simulink model "user_test"  (R2020a)
settings: Solver=VariableStepAuto  StartTime=0.0  StopTime=90  RelTol=1e-3
values from neighbouring files (symbols this model uses):
  r = r0    (= 1)    [get_LQR_gain.m]
undefined symbols (not defined in the file or in its folder): DiscIntNeverNeededParam, dt
settings Model: Creator=parke  LastModifiedBy=parke
settings SFSimCC: CustomCodeUndefinedFunction=UseInterfaceOnly

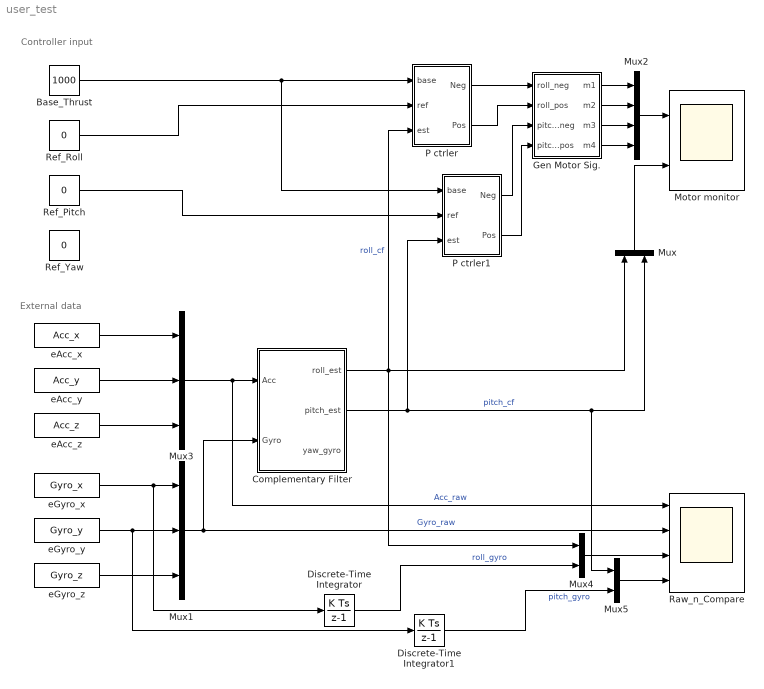
== system user_test ==
  note: External data
  note: Controller input
  Base_Thrust : Constant  Value=1000
  Complementary Filter : Subsystem
  Discrete-Time Integrator : DiscreteIntegrator  gainval=1  SampleTime=dt  ICPrevOutput=DiscIntNeverNeededParam  ICPrevScaledInput=DiscIntNeverNeededParam
  Discrete-Time Integrator1 : DiscreteIntegrator  gainval=1  SampleTime=dt  ICPrevOutput=DiscIntNeverNeededParam  ICPrevScaledInput=DiscIntNeverNeededParam
  Gen Motor Sig. : Subsystem
  Motor monitor : Scope  NumInputPorts=2
  Mux : Mux  Inputs=2
  Mux1 : Mux  Inputs=3
  Mux2 : Mux
  Mux3 : Mux  Inputs=3
  Mux4 : Mux  Inputs=2
  Mux5 : Mux  Inputs=2
  P ctrler : Subsystem
  P ctrler1 : Subsystem
  Raw_n_Compare : Scope  NumInputPorts=4
  Ref_Pitch : Constant  Value=0
  Ref_Roll : Constant  Value=0
  Ref_Yaw : Constant  Value=0
  eAcc_x : FromWorkspace  VariableName=Acc_x
  eAcc_y : FromWorkspace  VariableName=Acc_y
  eAcc_z : FromWorkspace  VariableName=Acc_z
  eGyro_x : FromWorkspace  VariableName=Gyro_x
  eGyro_y : FromWorkspace  VariableName=Gyro_y
  eGyro_z : FromWorkspace  VariableName=Gyro_z
  wires:
  eAcc_x/1 -> Mux3/1
  eAcc_z/1 -> Mux3/3
  eAcc_y/1 -> Mux3/2
  eGyro_x/1 -> Discrete-Time Integrator/1, Mux1/1
  eGyro_y/1 -> Discrete-Time Integrator1/1, Mux1/2
  eGyro_z/1 -> Mux1/3
  Mux4/1 -> Raw_n_Compare/3
  Complementary Filter/1(roll_est) -> Mux4/1, Mux/1, P ctrler/3(est)  "roll_cf"
  Mux1/1 -> Raw_n_Compare/2, Complementary Filter/2(Gyro)  "Gyro_raw"
  Complementary Filter/2(pitch_est) -> Mux5/1, Mux/2, P ctrler1/3(est)  "pitch_cf"
  Discrete-Time Integrator1/1 -> Mux5/2  "pitch_gyro"
  Discrete-Time Integrator/1 -> Mux4/2  "roll_gyro"
  Mux5/1 -> Raw_n_Compare/4
  Mux3/1 -> Complementary Filter/1(Acc), Raw_n_Compare/1  "Acc_raw"
  Ref_Roll/1 -> P ctrler/2(ref)
  Base_Thrust/1 -> P ctrler1/1(base), P ctrler/1(base)
  Ref_Pitch/1 -> P ctrler1/2(ref)
  Mux/1 -> Motor monitor/2
  P ctrler/1(Neg) -> Gen Motor Sig./1(roll_neg)
  P ctrler/2(Pos) -> Gen Motor Sig./2(roll_pos)
  Gen Motor Sig./3(m3) -> Mux2/3
  Gen Motor Sig./4(m4) -> Mux2/4
  P ctrler1/1(Neg) -> Gen Motor Sig./3(pitch_neg)
  P ctrler1/2(Pos) -> Gen Motor Sig./4(pitch_pos)
  Gen Motor Sig./1(m1) -> Mux2/1
  Gen Motor Sig./2(m2) -> Mux2/2
  Mux2/1 -> Motor monitor/1

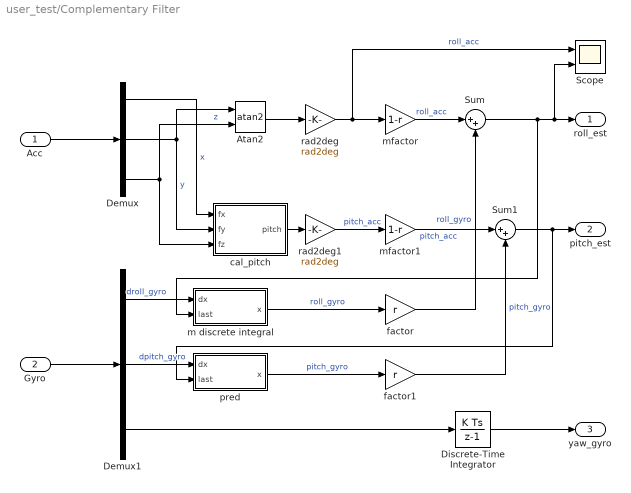
== system user_test/Complementary Filter ==
  Acc : Inport
  Gyro : Inport  Port=2
  Atan2 : Trigonometry  Operator=atan2
  Demux : Demux  Outputs=3
  Demux1 : Demux  Outputs=3
  Discrete-Time Integrator : DiscreteIntegrator  gainval=1  SampleTime=dt  ICPrevOutput=DiscIntNeverNeededParam  ICPrevScaledInput=DiscIntNeverNeededParam
  Scope : Scope  NumInputPorts=2
  Sum : Sum  Inputs=|++
  Sum1 : Sum  Inputs=|++
  cal_pitch : MATLAB Function  TreatAsAtomicUnit=on
  factor : Gain  Gain=r
  factor1 : Gain  Gain=r
  m discrete integral : Subsystem
  mfactor : Gain  Gain=1-r
  mfactor1 : Gain  Gain=1-r
  pred : Subsystem
  rad2deg : Gain  Gain=rad2deg
  rad2deg1 : Gain  Gain=rad2deg
  roll_est : Outport  VectorParamsAs1DForOutWhenUnconnected=off
  pitch_est : Outport  Port=2  VectorParamsAs1DForOutWhenUnconnected=off
  yaw_gyro : Outport  Port=3  VectorParamsAs1DForOutWhenUnconnected=off
  wires:
  Acc/1 -> Demux/1
  Gyro/1 -> Demux1/1
  Demux/2 -> cal_pitch/2(fy), Atan2/1  "y"
  Demux/3 -> cal_pitch/3(fz), Atan2/2  "z"
  Atan2/1 -> rad2deg/1
  Sum/1 -> m discrete integral/2(last), Scope/2, roll_est/1
  rad2deg/1 -> Scope/1, mfactor/1  "roll_acc"
  mfactor/1 -> Sum/1  "roll_acc"
  factor/1 -> Sum/2  "roll_gyro"
  Demux1/1 -> m discrete integral/1(dx)  "droll_gyro"
  m discrete integral/1(x) -> factor/1  "roll_gyro"
  Demux1/2 -> pred/1(dx)  "dpitch_gyro"
  pred/1(x) -> factor1/1  "pitch_gyro"
  Demux/1 -> cal_pitch/1(fx)  "x"
  Demux1/3 -> Discrete-Time Integrator/1
  Discrete-Time Integrator/1 -> yaw_gyro/1
  cal_pitch/1(pitch) -> rad2deg1/1
  rad2deg1/1 -> mfactor1/1  "pitch_acc"
  Sum1/1 -> pitch_est/1, pred/2(last)
  mfactor1/1 -> Sum1/1  "pitch_acc"
  factor1/1 -> Sum1/2  "pitch_gyro"

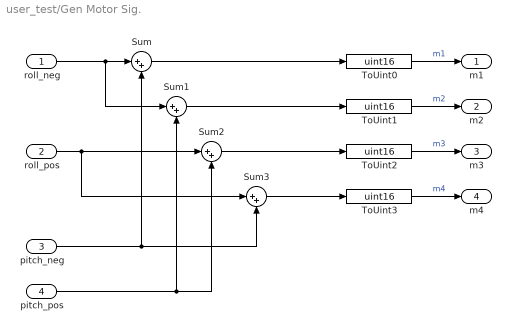
== system user_test/Gen Motor Sig. ==
  roll_neg : Inport
  roll_pos : Inport  Port=2
  pitch_neg : Inport  Port=3
  pitch_pos : Inport  Port=4
  Sum{,1..3} (4 alike) : Sum  Inputs=|++
  ToUint{0..3} (4 alike) : DataTypeConversion  OutDataTypeStr=uint16  SaturateOnIntegerOverflow=on
  m1 : Outport  VectorParamsAs1DForOutWhenUnconnected=off
  m2 : Outport  Port=2  VectorParamsAs1DForOutWhenUnconnected=off
  m3 : Outport  Port=3  VectorParamsAs1DForOutWhenUnconnected=off
  m4 : Outport  Port=4  VectorParamsAs1DForOutWhenUnconnected=off
  wires:
  ToUint2/1 -> m3/1  "m3"
  ToUint3/1 -> m4/1  "m4"
  ToUint1/1 -> m2/1  "m2"
  ToUint0/1 -> m1/1  "m1"
  roll_neg/1 -> Sum1/1, Sum/1
  pitch_neg/1 -> Sum/2, Sum3/2
  Sum/1 -> ToUint0/1
  pitch_pos/1 -> Sum1/2, Sum2/2
  Sum1/1 -> ToUint1/1
  Sum2/1 -> ToUint2/1
  roll_pos/1 -> Sum3/1, Sum2/1
  Sum3/1 -> ToUint3/1

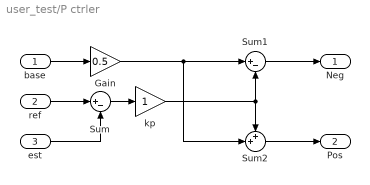
== system user_test/P ctrler ==
  base : Inport
  ref : Inport  Port=2
  est : Inport  Port=3
  Gain : Gain  Gain=0.5
  Sum : Sum  Inputs=|+-
  Sum1 : Sum  Inputs=|+-
  Sum2 : Sum  Inputs=++|
  kp : Gain
  Neg : Outport  VectorParamsAs1DForOutWhenUnconnected=off
  Pos : Outport  Port=2  VectorParamsAs1DForOutWhenUnconnected=off
  wires:
  base/1 -> Gain/1
  Sum1/1 -> Neg/1
  ref/1 -> Sum/1
  Sum/1 -> kp/1
  Sum2/1 -> Pos/1
  est/1 -> Sum/2
  kp/1 -> Sum1/2, Sum2/1
  Gain/1 -> Sum2/2, Sum1/1

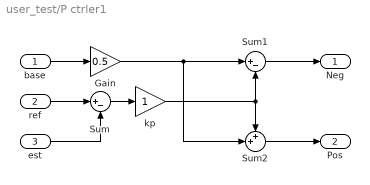
== system user_test/P ctrler1 ==
  base : Inport
  ref : Inport  Port=2
  est : Inport  Port=3
  Gain : Gain  Gain=0.5
  Sum : Sum  Inputs=|+-
  Sum1 : Sum  Inputs=|+-
  Sum2 : Sum  Inputs=++|
  kp : Gain
  Neg : Outport  VectorParamsAs1DForOutWhenUnconnected=off
  Pos : Outport  Port=2  VectorParamsAs1DForOutWhenUnconnected=off
  wires:
  base/1 -> Gain/1
  Sum1/1 -> Neg/1
  ref/1 -> Sum/1
  Sum/1 -> kp/1
  Sum2/1 -> Pos/1
  est/1 -> Sum/2
  kp/1 -> Sum1/2, Sum2/1
  Gain/1 -> Sum2/2, Sum1/1

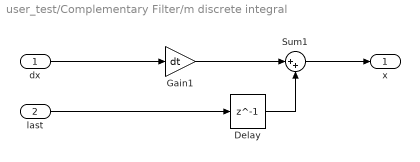
== system user_test/Complementary Filter/m discrete integral ==
  dx : Inport
  last : Inport  Port=2
  Delay : Delay  DelayLength=1  InitialCondition=0  SampleTime=dt
  Gain1 : Gain  Gain=dt
  Sum1 : Sum  Inputs=|++
  x : Outport  VectorParamsAs1DForOutWhenUnconnected=off
  wires:
  dx/1 -> Gain1/1
  Delay/1 -> Sum1/2
  last/1 -> Delay/1
  Sum1/1 -> x/1
  Gain1/1 -> Sum1/1

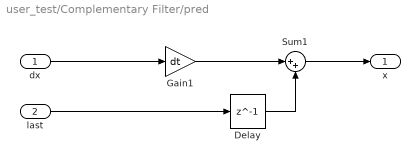
== system user_test/Complementary Filter/pred ==
  dx : Inport
  last : Inport  Port=2
  Delay : Delay  DelayLength=1  InitialCondition=0  SampleTime=dt
  Gain1 : Gain  Gain=dt
  Sum1 : Sum  Inputs=|++
  x : Outport  VectorParamsAs1DForOutWhenUnconnected=off
  wires:
  dx/1 -> Gain1/1
  Delay/1 -> Sum1/2
  last/1 -> Delay/1
  Sum1/1 -> x/1
  Gain1/1 -> Sum1/1

== matlab function user_test/Complementary Filter/cal_pitch ==
  data: fx input; pitch output; fy input; fz input
function pitch = fcn(fx, fy, fz)

pitch = atan2(-fx,norm([fy,fz]));
